simulink model "GazeboDifferentialDriveControl"  (R2021a)
settings: Solver=FixedStepAuto  StartTime=0.0  StopTime=15  RelTol=1e-3
StopFcn:
  | robotPoses = out.yout{1}.Values.Data;
  | 
  | figure;
  | plot(wayPoints(:,1), wayPoints(:,2), 'k-x');
  | hold all
  | plot(robotPoses(:,1), robotPoses(:,2));
  | title('XY Waypoint Tracking');
values from neighbouring files (symbols this model uses):
  odom = rossubscriber('/odom')    [trialRRT_with_control_iterative.m]
  wayPoints = wayPoints - 50    [trialRRT_with_control_iterative.m]
undefined symbols (not defined in the file or in its folder): Angular, Linear
libraries: robotlib x4, robotgazebolib x4, robotalgslib x1, robotcorelib x1, simulink x1
settings Model: PacingRate=0.011000  OrderedModelArguments=off  Creator=The MathWorks, Inc.  LastModifiedBy=sskulka
settings SolverCC: AlgebraicLoopSolver=TrustRegion
settings OptimizationCC: EnhancedBackFolding=on  PassReuseOutputArgsAs=Individual arguments  ZeroExternalMemoryAtStartup=off  ZeroInternalMemoryAtStartup=off  MaxStackSize=64  OptimizeBlockOrder=speed  DifferentSizesBufferReuse=on  OptimizationCustomize=off  EfficientTunableParamExpr=on
settings DebuggingCC: ParameterTunabilityLossMsg=error  SymbolicDimsDataTypeCodeGenerationDiagnostic=none  SFMachineParentedDataDiag=warning
settings HardwareCC: ProdBitPerPointer=32  ProdBitPerSizeT=32  ProdBitPerPtrDiffT=32  ProdLargestAtomicFloat=None  ProdIntDivRoundTo=Undefined  ProdEndianess=Unspecified  ProdWordSize=32  ProdHWDeviceType=Generic->Unspecified (assume 32-bit Generic)
settings SFSimCC: MATLABDynamicMemAlloc=off
settings RTWCC: SystemTargetFile=ert.tlc  HardwareBoard=Robot Operating System (ROS)  TLCOptions="-aInlineSetEventsForThisBaseRateFcn=TLC_FALSE -aSuppressMultiTaskScheduler=TLC_FALSE  -aRateBasedStepFcn=0"  TemplateMakefile=ert_default_tmf  Toolchain=Catkin  TargetLang=C++
settings CodeAppCC: ForceParamTrailComments=on  IgnoreCustomStorageClasses=off  OperatorAnnotations=on  SimulinkDataObjDesc=on  SFDataObjDesc=on  InsertBlockDesc=on

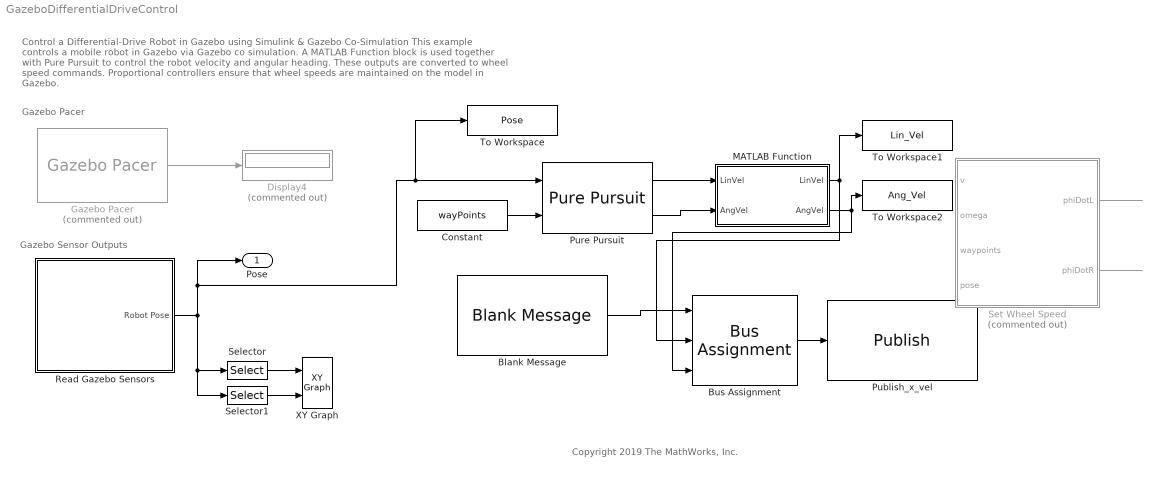
== system GazeboDifferentialDriveControl ==
  note: Gazebo Pacer
  note: Control a Differential-Drive Robot in Gazebo using Simulink & Gazebo Co-Simulation
      | This example controls a mobile robot in Gazebo via Gazebo co simulation. A MATLAB Function block is used together with Pure Pursuit to control the robot velocity and angular heading. These outputs are converted to wheel speed commands. Proportional controllers ensure that wheel speeds are maintained on the model in Gazebo.
  note: Copyright 2019 The MathWorks, Inc.
  note: Gazebo Sensor Outputs
  Blank Message : robotlib/Blank Message  messageClass=Message  entityType=geometry_msgs/Twist  messageType=geometry_msgs/Twist  SampleTime=inf  legacyBusStruct=off
  Bus Assignment : BusAssignment  AssignedSignals=Linear.X,Angular.Z
  Constant : Constant  Value=wayPoints
  Display4 : Display  Commented=on
  Gazebo Pacer : robotgazebolib/Gazebo Pacer  Commented=on  ResetBehavior=Reset Gazebo simulation time and scene  SampleTime=0.01
      settings: SourceProductBaseCode=RO
  MATLAB Function : MATLAB Function  TreatAsAtomicUnit=on
  Publish_x_vel : robotlib/Publish  topicSource=Select from ROS network  topic=/cmd_vel  messageType=geometry_msgs/Twist  legacyBusStruct=off  messageQueueLength=1
  Pure Pursuit : robotalgslib/Pure Pursuit  DesiredLinearVelocity=1  MaxAngularVelocity=1.0  LookaheadDistance=1.0  TargetDirPort=off  SimulateUsing=Code generation
  Read Gazebo Sensors : Subsystem
  Selector : Selector  InputPortWidth=3  IndexOptions=Index vector (dialog)  Indices=[1]  OutputSizes=1
  Selector1 : Selector  InputPortWidth=3  IndexOptions=Index vector (dialog)  Indices=[2]  OutputSizes=1
  Set Wheel Speed : MATLAB Function  Commented=on  TreatAsAtomicUnit=on
  To Workspace : ToWorkspace  VariableName=Pose  SampleTime=-1
  To Workspace1 : ToWorkspace  VariableName=Lin_Vel  SampleTime=-1
  To Workspace2 : ToWorkspace  VariableName=Ang_Vel  SampleTime=-1
  XY Graph : simulink/Sinks/XY Graph  xmin=-3  xmax=4  ymin=-1  ymax=8  st=-1
  Pose : Outport
  wires:
  Set Wheel Speed/1(phiDotL) -> ?
  Gazebo Pacer/1 -> Display4/1
  Constant/1 -> Pure Pursuit/2
  Read Gazebo Sensors/1(Robot Pose) -> Pose/1, To Workspace/1, Pure Pursuit/1, Selector/1, Selector1/1
  Selector/1 -> XY Graph/1
  Selector1/1 -> XY Graph/2
  Pure Pursuit/1 -> MATLAB Function/1("LinVel ")
  Set Wheel Speed/2(phiDotR) -> ?
  Blank Message/1 -> Bus Assignment/1
  Bus Assignment/1 -> Publish_x_vel/1
  Pure Pursuit/2 -> MATLAB Function/2("AngVel ")
  MATLAB Function/1(LinVel) -> Bus Assignment/2, To Workspace1/1
  MATLAB Function/2(AngVel) -> Bus Assignment/3, To Workspace2/1

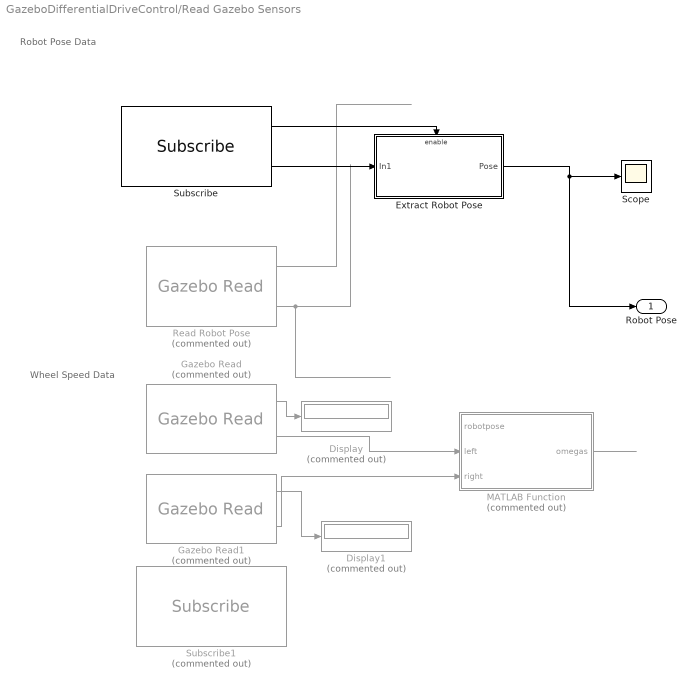
== system GazeboDifferentialDriveControl/Read Gazebo Sensors ==
  note: Robot Pose Data
  note: Wheel Speed Data
  Display : Display  Commented=on
  Display1 : Display  Commented=on
  Extract Robot Pose : Subsystem
  Gazebo Read : robotgazebolib/Gazebo Read  Commented=on  topicSource=From Gazebo  topic=/gazebo/ground_truth/world_pose/pioneer2dx/left_wheel  messageType=gazebo_msgs/Pose  sampleTime=0.01
      settings: SourceProductBaseCode=RO
  Gazebo Read1 : robotgazebolib/Gazebo Read  Commented=on  topicSource=From Gazebo  topic=/gazebo/ground_truth/world_pose/pioneer2dx/right_wheel  messageType=gazebo_msgs/Pose  sampleTime=0.01
      settings: SourceProductBaseCode=RO
  MATLAB Function : MATLAB Function  Commented=on  TreatAsAtomicUnit=on
  Read Robot Pose : robotgazebolib/Gazebo Read  Commented=on  topicSource=Specify your own  topic=/odom  messageType=gazebo_msgs/Pose  sampleTime=0.01
      settings: SourceProductBaseCode=RO
  Scope : Scope
  Subscribe : robotlib/Subscribe  topicSource=Select from ROS network  topic=/odom  messageType=nav_msgs/Odometry  SampleTime=-1  legacyBusStruct=off  messageQueueLength=1
  Subscribe1 : robotlib/Subscribe  Commented=on  topicSource=Select from ROS network  topic=/gazebo/link_states  messageType=gazebo_msgs/LinkStates  SampleTime=-1  legacyBusStruct=off  messageQueueLength=1
  Robot Pose : Outport
  wires:
  Read Robot Pose/2 -> ?
  Extract Robot Pose/1(Pose) -> Scope/1, Robot Pose/1
  Read Robot Pose/1 -> ?
  Gazebo Read/1 -> Display/1
  Gazebo Read1/1 -> Display1/1
  MATLAB Function/1(omegas) -> ?
  Gazebo Read/2 -> MATLAB Function/2(left)
  Gazebo Read1/2 -> MATLAB Function/3(right)
  Subscribe/2 -> Extract Robot Pose/1(In1)
  Subscribe/1 -> Extract Robot Pose/Enable

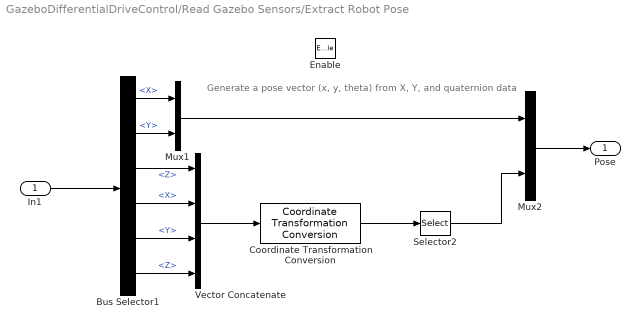
== system GazeboDifferentialDriveControl/Read Gazebo Sensors/Extract Robot Pose ==
  note: Generate a pose vector (x, y, theta) from X, Y, and quaternion data
  In1 : Inport
  Enable : EnablePort
  Bus Selector1 : BusSelector  OutputSignals=Twist.Twist.Linear.X,Twist.Twist.Linear.Y,Twist.Twist.Linear.Z,Twist.Twist.Angular.X,Twist.Twist.Angular.Y,Twist.Twist.Angular.Z
  Coordinate Transformation Conversion : robotcorelib/Coordinate Transformation Conversion  InputRepresentation=Quaternion  InputEulerSequence=ZYX  ShowTrVecInputPort=on  OutputRepresentation=Euler Angles  OutputEulerSequence=ZYX  ShowTrVecOutputPort=on  SimulateUsing=Interpreted execution
      settings: SourceProductBaseCode=NV,RO,RR,UV
  Mux1 : Mux  Inputs=2
  Mux2 : Mux  Inputs=2
  Selector2 : Selector  InputPortWidth=3  IndexOptions=Index vector (dialog)  Indices=1  OutputSizes=1
  Vector Concatenate : Concatenate  NumInputs=4
  Pose : Outport  VectorParamsAs1DForOutWhenUnconnected=off
  wires:
  Vector Concatenate/1 -> Coordinate Transformation Conversion/1
  Coordinate Transformation Conversion/1 -> Selector2/1
  Mux1/1 -> Mux2/1
  Selector2/1 -> Mux2/2
  Mux2/1 -> Pose/1
  Bus Selector1/6 -> Vector Concatenate/4  "<Z>"
  Bus Selector1/1 -> Mux1/1  "<X>"
  Bus Selector1/4 -> Vector Concatenate/2  "<X>"
  Bus Selector1/2 -> Mux1/2  "<Y>"
  Bus Selector1/3 -> Vector Concatenate/1  "<Z>"
  Bus Selector1/5 -> Vector Concatenate/3  "<Y>"
  In1/1 -> Bus Selector1/1

== matlab function GazeboDifferentialDriveControl/Read Gazebo Sensors/MATLAB Function ==
  data: robotpose input; omegas output; left input; right input
function omegas = computeWheelVelocities(robotpose, left, right)
%computeWheelVelocities computes wheel velocity based on rate of change of
%the yaw angle of the wheel relative to its original mount on the robot
%body

persistent initAngles
if isempty(initAngles)
    initAngles = zeros(2,1);
end
sampleTime = 0.01;

% compute rotation between wheel original mount on the robot body and world
% frame
robotRtom = quat2rotm([robotpose.orientation.w, robotpose.orientation.x, robotpose.orientation.y, robotpose.orientation.z]);
originalWheelMount = robotRtom*eul2rotm([pi/2 pi/2 0]);

% get rotation between wheel and the world frame
leftRtom = quat2rotm([left.orientation.w, left.orientation.x, left.orientation.y, left.orientation.z]);
rightRtom = quat2rotm([right.orientation.w, right.orientation.x, right.orientation.y, right.orientation.z]);

% compute relative rotation between wheel and its original mount
leftRotation = rotm2eul(originalWheelMount'*leftRtom);
rightRotation = rotm2eul(originalWheelMount'*rightRtom);

% compute angluar velocity using the angle difference between the current
% angle pose and the the angle pose in last time step
angles = [leftRotation(1); rightRotation(1)];
omegas = angdiff(initAngles, angles)/sampleTime;
initAngles = angles;

== matlab function GazeboDifferentialDriveControl/Set Wheel Speed ==
  data: v input; omega input; waypoints input; pose input; phiDotL output; phiDotR output
function [phiDotL, phiDotR] = wheelSpeed(v, omega, waypoints, pose)

% Path constants
stopThreshold = 0.1;
slowThreshold = 0.3;

% Robot constants
trackWidth = 0.381;
wheelRadius = 0.195/2;

% Slow the robot down when it's near the threshold
distanceToEndpoint = norm(waypoints(end, :) - pose(1:2)');
if (distanceToEndpoint < slowThreshold)
    v = distanceToEndpoint/slowThreshold*v;
    
    % Stop the robot if it's inside the target threshold
    if distanceToEndpoint < stopThreshold
        v = 0;
    end
end

% Convert velocity and heading angular velocity to wheel speeds
phiDotL = (v - trackWidth/2*omega)/wheelRadius;
phiDotR = (v + trackWidth/2*omega)/wheelRadius;

end

== matlab function GazeboDifferentialDriveControl/MATLAB Function ==
  data: LinVel input; LinVel output; AngVel input; AngVel output
function [LinVel, AngVel] = fcn(LinVel, AngVel)
if(LinVel > 0 || LinVel < -1)
    LinVel = LinVel;
    AngVel = AngVel;
else
    LinVel = 0;
    AngVel = 0;
end    
%y = u;
